simulink model "VGrowth3"  (R2018b)
settings: Solver=VariableStepAuto  StartTime=0  StopTime=20  RelTol=1e-3
libraries: nesl_utility x4, sh_lib x3, fl_lib x1, sdl_lib x1
settings Model: Creator=Magneto  LastModifiedBy=Magneto

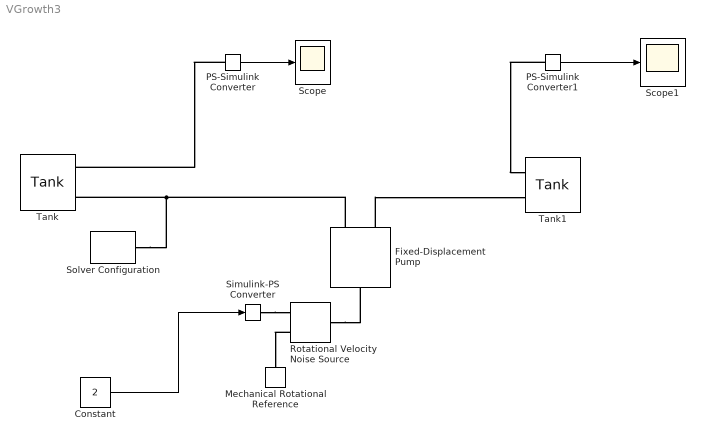
== system VGrowth3 ==
  Constant : Constant  Value=2
  Fixed-Displacement Pump : sh_lib/Pumps and Motors/Fixed-Displacement Pump  D=30 cm^3/rev  loss_spec=1  w_nominal=188 rad/s  pr_nominal=100e5 Pa  visc_nominal=18 cSt  dens_nominal=900 kg/m^3  efficiency_vol=0.92  no_load_torque=0.05 N*m  torque_pressure_coeff=0.6e-6 N*m/Pa  p_diff_eff_TLU=[100000, 1000000, 2000000] Pa  omega_eff_TLU=[25, 50, 100, 200, 300, 400] rad/s  vol_eff_TLU=[.816, .908, .954, .977, .981, .984; .325, .663, .831, .916, .925, .946; .137, .568, .78, .892, .893, .91]  mech_eff_TLU=[.996, .996, .996, .996, .996, .996; .988, .989, .989, .989, .989, .99; .981, .981, .982, .982, .983, .984]  p_diff_loss_TLU=[100000, 1000000, 2000000] Pa  omega_loss_TLU=[25, 50, 100, 200, 300, 400] rad/s  vol_loss_TLU=[.023, .023, .023, .023, .0285, .032; .0844, .0842, .0845, .084, .1125, .108; .1079, .108, .11, .108, .1605, .18] * 1e-3 m^3/s  mech_loss_TLU=[.002, .002, .002, .002, .002, .002; .0607, .0556, .0556, .0556, .0556, .0505; .1937, .1937, .1833, .1833, .1729, .1626] N*m  pressure_threshold=1e5 Pa  omega_threshold=10 rad/s  quadrant_check=0  pressure_check=0  min_valid_pressure=0 Pa  vol_eff_min=1e-3  vol_eff_max=1  mech_eff_min=1e-3  mech_eff_max=1
      settings: SourceProductName=Simscape Fluids  SourceProductBaseCode=SH
  Mechanical Rotational Reference : fl_lib/Mechanical/Rotational Elements/Mechanical Rotational Reference
  PS-Simulink Converter : nesl_utility/PS-Simulink Converter  PhysicalDomain=network_engine_domain  SubClassName=ps_output  LeftPortType=input  RightPortType=output  PseudoPeriodic=off  Frequencies=[]  Unit=1  AffineConversion=off
  PS-Simulink Converter1 : nesl_utility/PS-Simulink Converter  PhysicalDomain=network_engine_domain  SubClassName=ps_output  LeftPortType=input  RightPortType=output  PseudoPeriodic=off  Frequencies=[]  Unit=1  AffineConversion=off
  Rotational Velocity Noise Source : sdl_lib/Sources/Rotational Velocity Noise Source  sample_time=1e-3 s  repeatability=1  user_seed=0  auto_seed=2730683129
      settings: SourceProductName=Simscape Driveline  SourceProductBaseCode=LD
  Scope : Scope
  Scope1 : Scope
  Simulink-PS Converter : nesl_utility/Simulink-PS Converter  PhysicalDomain=network_engine_domain  SubClassName=ps_input  LeftPortType=input  RightPortType=output  PseudoPeriodic=off  Frequencies=[]  NoiseDistribution=none  NoiseParameters=[]  Unit=1  AffineConversion=off  FilteringAndDerivatives=provide  SimscapeFilterOrder=1  InputFilterTimeConstant=0.001  UdotUserProvided=0
  Solver Configuration : nesl_utility/Solver Configuration  PhysicalDomain=network_engine_domain  SubClassName=solver  LeftPortType=input  RightPortType=generic  Tones=[]  Harmonics=[]  SimulateNoise=off  Profile=off  UseLocalSampling=off  EnableSwitchedLinearOptims=on  FrequencyDomain=off  UseCCode=off  RelTol=0.001  AbsTol=1e-06  MinStep=1e-09  ToWorkspace=off  RevertToSquareIcSolve=off  NumHomotopyIterations=100  PhasorMode=off  PhasorModeNumHarmonics=1  DoDC=off  ResidualTolerance=1e-09  UseLocalSolver=off  LocalSolverChoice=NE_BACKWARD_EULER_ADVANCER  LocalSolverSampleTime=0.001  DoFixedCost=off  MaxNonlinIter=3  MaxModeIter=2  LinearAlgebra=auto  EquationFormulation=NE_TIME_EF  DelaysMemoryBudget=1024  AutomaticFiltering=on  FilteringTimeConstant=0.001  PartitionStorageMethod=AS_NEEDED  PartitionMemoryBudget=1024
  Tank : sh_lib/Low-Pressure Blocks/Tank  press=0 Pa  level_spec=1  tank_area=0.8 m^2  fluid_volume_tab=[0, .0028, .0065, .0114, .0176, .0252, .0344, .0436, .0512, .0574, .0623, .066, .0688, .0707, .072, .0727] m^3  fluid_level_tab=[0, .02, .04, .06, .08, .1, .12, .14, .16, .18, .2, .22, .24, .26, .28, .3] m  interp_method=1  extrap_method=1  pipe_diam=0.02 m  loss_coeff=1.2  g=9.80665 m/s^2  min_level=1e-3 m  fluid_level_check=0  volume_specify=on  volume_priority=High  volume=2.78e9 l  volume_nominal_specify=off  volume_nominal_unit=l  volume_nominal_value=1  level_specify=off  level_priority=None  level=0.025 m  level_nominal_specify=off  level_nominal_unit=m  level_nominal_value=1  pipe_diam_A=0.02 m  loss_coeff_A=1.2  height_B=0.8 m  pipe_diam_B=0.02 m  loss_coeff_B=1.2  height_C=0.8 m  pipe_diam_C=0.02 m  loss_coeff_C=1.2
      settings: SourceProductName=Simscape Fluids  SourceProductBaseCode=SH
  Tank1 : sh_lib/Low-Pressure Blocks/Tank  press=0 Pa  level_spec=1  tank_area=0.8 m^2  fluid_volume_tab=[0, .0028, .0065, .0114, .0176, .0252, .0344, .0436, .0512, .0574, .0623, .066, .0688, .0707, .072, .0727] m^3  fluid_level_tab=[0, .02, .04, .06, .08, .1, .12, .14, .16, .18, .2, .22, .24, .26, .28, .3] m  interp_method=1  extrap_method=1  pipe_diam=0.02 m  loss_coeff=1.2  g=9.80665 m/s^2  min_level=1e-3 m  fluid_level_check=0  volume_specify=on  volume_priority=High  volume=0 l  volume_nominal_specify=off  volume_nominal_unit=l  volume_nominal_value=1  level_specify=off  level_priority=None  level=0.025 m  level_nominal_specify=off  level_nominal_unit=m  level_nominal_value=1  pipe_diam_A=0.02 m  loss_coeff_A=1.2  height_B=0.8 m  pipe_diam_B=0.02 m  loss_coeff_B=1.2  height_C=0.8 m  pipe_diam_C=0.02 m  loss_coeff_C=1.2
      settings: SourceProductName=Simscape Fluids  SourceProductBaseCode=SH
  wires:
  PS-Simulink Converter/1 -> Scope/1
  PS-Simulink Converter1/1 -> Scope1/1
  Constant/1 -> Simulink-PS Converter/1
  connections:
  Fixed-Displacement Pump/RConn1 -- Solver Configuration/RConn1 -- Tank/RConn2
  Fixed-Displacement Pump/RConn2 -- Tank1/RConn2
  Rotational Velocity Noise Source/RConn1 -- Fixed-Displacement Pump/LConn1
  Rotational Velocity Noise Source/LConn2 -- Mechanical Rotational Reference/LConn1
  PS-Simulink Converter/LConn1 -- Tank/RConn1
  PS-Simulink Converter1/LConn1 -- Tank1/RConn1
  Simulink-PS Converter/RConn1 -- Rotational Velocity Noise Source/LConn1
